simulink model "P2001_230205_InstantaneousCostAnalysis1"  (R2022b)
settings: Solver=VariableStepAuto  StartTime=0.0  StopTime=10  RelTol=1e-6
settings Model: Creator=turib  LastModifiedBy=turib

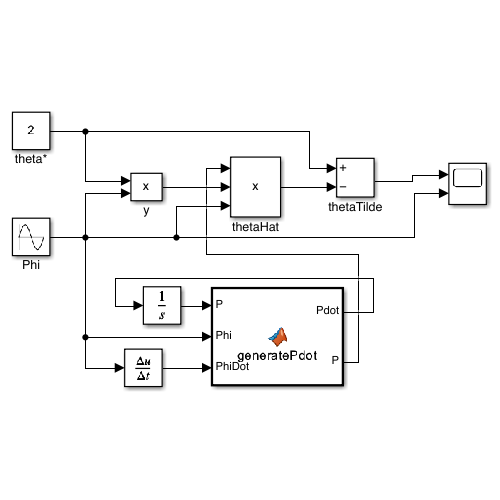
[thumbnail: Simulink's stored preview of the top-level diagram]
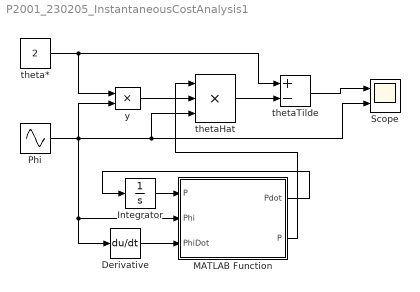
== system P2001_230205_InstantaneousCostAnalysis1 ==
  Derivative : Derivative
  Integrator : Integrator
  MATLAB Function : MATLAB Function  TreatAsAtomicUnit=on
  Phi : Sin  SampleTime=0
  Scope : Scope  NumInputPorts=2
  theta* : Constant  Value=2
  thetaHat : Product  Inputs=3
  thetaTilde : Sum  Inputs=+-
  y : Product
  wires:
  Phi/1 -> Scope/2, thetaHat/3, MATLAB Function/2(Phi), Derivative/1, y/2
  theta*/1 -> thetaTilde/1, y/1
  Derivative/1 -> MATLAB Function/3(PhiDot)
  MATLAB Function/1(Pdot) -> Integrator/1
  Integrator/1 -> MATLAB Function/1("P ")
  y/1 -> thetaHat/2
  MATLAB Function/2(P) -> thetaHat/1
  thetaHat/1 -> thetaTilde/2
  thetaTilde/1 -> Scope/1

== matlab function P2001_230205_InstantaneousCostAnalysis1/MATLAB Function ==
  data: Pdot output; P output; P input; Phi input; PhiDot input
function [Pdot, P] = generatePdot(P, Phi, PhiDot)

Pdot = -2 * P ^ 2 * Phi * PhiDot;

end
